simulink model "RadarAltimeter"  (R2020b)
settings: Solver=FixedStepAuto  StartTime=0.0  StopTime=0.0001  FixedStep=T_step  RelTol=1e-3
values from neighbouring files (symbols this model uses):
  BPFden = [RH*RL*CH*CL,RH*CH+RL*CL,1]    [RadarAltEval2.m]
  BPFnum = [RH*CH,0]    [RadarAltEval2.m]
  f_carrier = 1e9    (= 1000000000)    [RadarAltEval.m]    (also in RadarAltEval2.m = 450000000)
  f_square = 500000    [RadarAltEval.m]    (also in RadarAltEval2.m = 250000)
  FMgain = 5    [RadarAltEval.m]    (also in RadarAltEval2.m)
  h = 20    [RadarAltEval.m]    (also in RadarAltEval2.m = 80)
  k_VCO = 2*BW/V_square    (= 200)    [RadarAltEval.m]    (also in RadarAltEval2.m = 400)
  LPFden = conv(LPFden,LPFden)    [RadarAltEval2.m]
  LPFnum = 1    [RadarAltEval2.m]
  noiseVar = 0    [RadarAltEval.m]    (also in RadarAltEval2.m)
  RXdir = 1.76    [RadarAltEval.m]    (also in RadarAltEval2.m)
  RXnoiseVar = 0    [RadarAltEval.m]    (also in RadarAltEval2.m)
  speed = 0    [RadarAltEval.m]    (also in RadarAltEval2.m)
  TXdir = 1.76    [RadarAltEval.m]    (also in RadarAltEval2.m)
  V_square = 10    [RadarAltEval.m]    (also in RadarAltEval2.m)
undefined symbols (not defined in the file or in its folder): magnitude
settings Model: Creator=Joseph  LastModifiedBy=Joseph

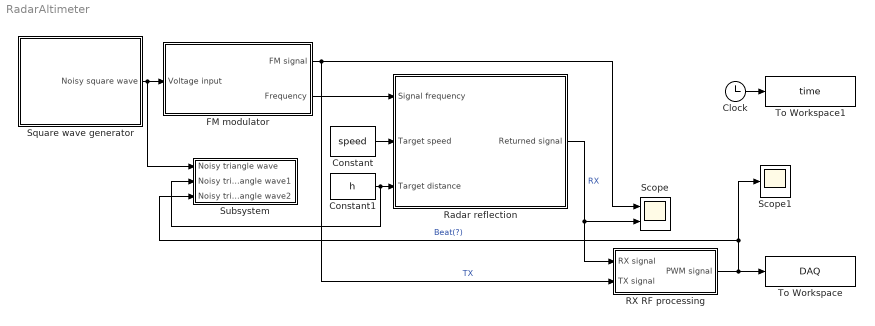
== system RadarAltimeter ==
  Clock : Clock
  Constant : Constant  Value=speed
  Constant1 : Constant  Value=h
  FM modulator : Subsystem
  RX RF processing : Subsystem
  Radar reflection : Subsystem
  Scope : Scope  NumInputPorts=2
  Scope1 : Scope
  Square wave generator : Subsystem
  Subsystem : Subsystem
  To Workspace : ToWorkspace  VariableName=DAQ  SampleTime=-1
  To Workspace1 : ToWorkspace  VariableName=time  SampleTime=-1
  wires:
  Square wave generator/1(Noisy square wave) -> Subsystem/1(Noisy triangle wave), FM modulator/1(Voltage input)
  FM modulator/1(FM signal) -> RX RF processing/2(TX signal), Scope/1  "TX"
  Radar reflection/1(Returned signal) -> RX RF processing/1(RX signal), Scope/2  "RX"
  FM modulator/2(Frequency) -> Radar reflection/1(Signal frequency)
  Constant/1 -> Radar reflection/2(Target speed)
  Constant1/1 -> Subsystem/2(Noisy triangle wave1), Radar reflection/3(Target distance)
  RX RF processing/1(PWM signal) -> Subsystem/3(Noisy triangle wave2), Scope1/1, To Workspace/1  "Beat(?)"
  Clock/1 -> To Workspace1/1

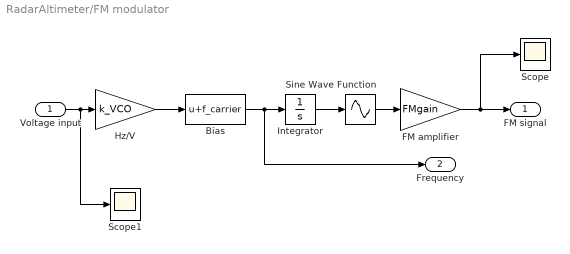
== system RadarAltimeter/FM modulator ==
  Voltage input : Inport
  Bias : Bias  Bias=f_carrier
  FM amplifier : Gain  Gain=FMgain
  Hz/V : Gain  Gain=k_VCO
  Integrator : Integrator
  Scope : Scope
  Scope1 : Scope
  Sine Wave Function : Sin  TimeSource=Use external signal  Frequency=2*pi  SampleTime=0
  FM signal : Outport
  Frequency : Outport  Port=2
  wires:
  Voltage input/1 -> Scope1/1, Hz/V/1
  Sine Wave Function/1 -> FM amplifier/1
  Bias/1 -> Frequency/1, Integrator/1
  Hz/V/1 -> Bias/1
  Integrator/1 -> Sine Wave Function/1
  FM amplifier/1 -> Scope/1, FM signal/1

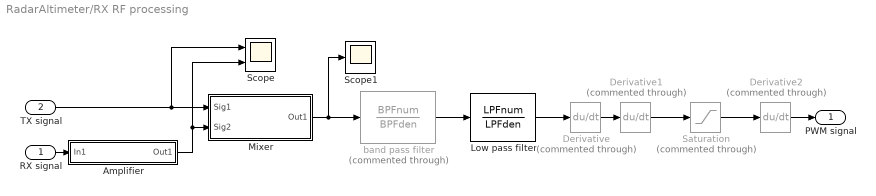
== system RadarAltimeter/RX RF processing ==
  RX signal : Inport
  TX signal : Inport  Port=2
  Amplifier : Subsystem
  Derivative : Derivative  Commented=through
  Derivative1 : Derivative  Commented=through
  Derivative2 : Derivative  Commented=through
  Low pass filter : TransferFcn  Numerator=LPFnum  Denominator=LPFden
  Mixer : Subsystem
  Saturation : Saturate  Commented=through  UpperLimit=3  LowerLimit=0
  Scope : Scope  NumInputPorts=2
  Scope1 : Scope
  band pass filter : TransferFcn  Commented=through  Numerator=BPFnum  Denominator=BPFden
  PWM signal : Outport
  wires:
  TX signal/1 -> Mixer/1(Sig1), Scope/1
  Mixer/1(Out1) -> band pass filter/1, Scope1/1
  Amplifier/1(Out1) -> Scope/2, Mixer/2(Sig2)
  RX signal/1 -> Amplifier/1(In1)
  Derivative/1 -> Derivative1/1
  band pass filter/1 -> Low pass filter/1
  Low pass filter/1 -> Derivative/1
  Saturation/1 -> Derivative2/1
  Derivative1/1 -> Saturation/1
  Derivative2/1 -> PWM signal/1

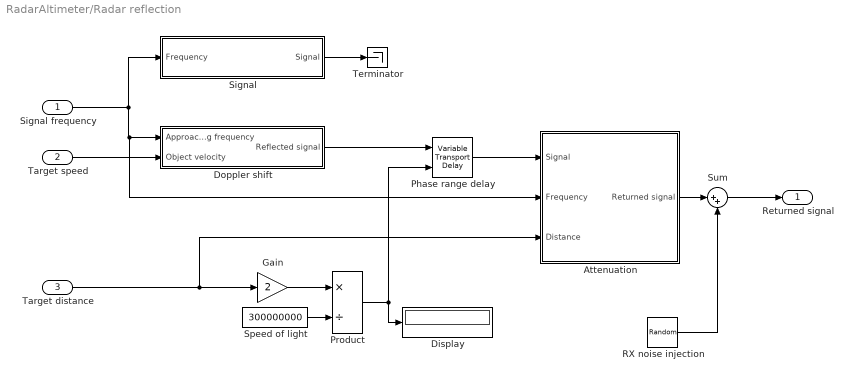
== system RadarAltimeter/Radar reflection ==
  Signal frequency : Inport
  Target speed : Inport  Port=2
  Target distance : Inport  Port=3
  Attenuation : Subsystem
  Display : Display
  Doppler shift : Subsystem
  Gain : Gain  Gain=2
  Phase range delay : VariableTransportDelay  MaximumDelay=10
  Product : Product  Inputs=*/
  RX noise injection : RandomNumber  Variance=RXnoiseVar  Seed=randi([0,10000])  SampleTime=0.1
  Signal : Subsystem
  Speed of light : Constant  Value=300000000
  Sum : Sum  Inputs=|++
  Terminator : Terminator
  Returned signal : Outport
  wires:
  Sum/1 -> Returned signal/1
  Doppler shift/1(Reflected signal) -> Phase range delay/1
  Phase range delay/1 -> Attenuation/1(Signal)
  Signal frequency/1 -> Attenuation/2(Frequency), Doppler shift/1(Approaching frequency), Signal/1(Frequency)
  Gain/1 -> Product/1
  Speed of light/1 -> Product/2
  Product/1 -> Display/1, Phase range delay/2
  Target distance/1 -> Attenuation/3(Distance), Gain/1
  Target speed/1 -> Doppler shift/2(Object velocity)
  Attenuation/1(Returned signal) -> Sum/1
  RX noise injection/1 -> Sum/2
  Signal/1(Signal) -> Terminator/1

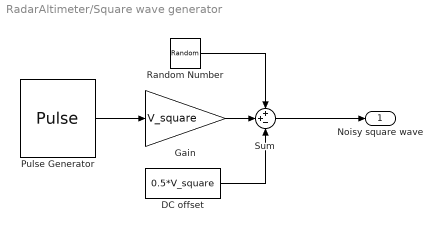
== system RadarAltimeter/Square wave generator ==
  DC offset : Constant  Value=0.5*V_square
  Gain : Gain  Gain=V_square
  Pulse Generator : DiscretePulseGenerator  PulseType=Time based  Period=1/f_square  PulseWidth=50
  Random Number : RandomNumber  Variance=noiseVar  Seed=randi([0,10000])
  Sum : Sum  Inputs=++-
  Noisy square wave : Outport
  wires:
  Pulse Generator/1 -> Gain/1
  Gain/1 -> Sum/2
  DC offset/1 -> Sum/3
  Sum/1 -> Noisy square wave/1
  Random Number/1 -> Sum/1

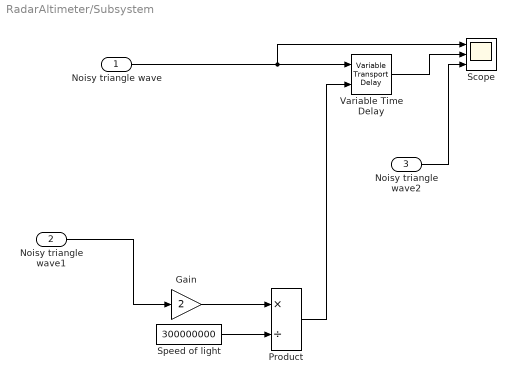
== system RadarAltimeter/Subsystem ==
  Noisy triangle wave : Inport
  Noisy triangle wave1 : Inport  Port=2
  Noisy triangle wave2 : Inport  Port=3
  Gain : Gain  Gain=2
  Product : Product  Inputs=*/
  Scope : Scope  NumInputPorts=3
  Speed of light : Constant  Value=300000000
  Variable Time Delay : VariableTransportDelay  MaximumDelay=10
  wires:
  Noisy triangle wave/1 -> Scope/1, Variable Time Delay/1
  Gain/1 -> Product/1
  Noisy triangle wave1/1 -> Gain/1
  Speed of light/1 -> Product/2
  Product/1 -> Variable Time Delay/2
  Variable Time Delay/1 -> Scope/2
  Noisy triangle wave2/1 -> Scope/3

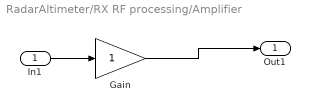
== system RadarAltimeter/RX RF processing/Amplifier ==
  In1 : Inport
  Gain : Gain
  Out1 : Outport
  wires:
  In1/1 -> Gain/1
  Gain/1 -> Out1/1

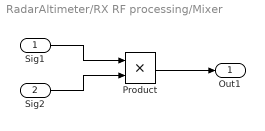
== system RadarAltimeter/RX RF processing/Mixer ==
  Sig1 : Inport
  Sig2 : Inport  Port=2
  Product : Product
  Out1 : Outport
  wires:
  Sig1/1 -> Product/1
  Sig2/1 -> Product/2
  Product/1 -> Out1/1

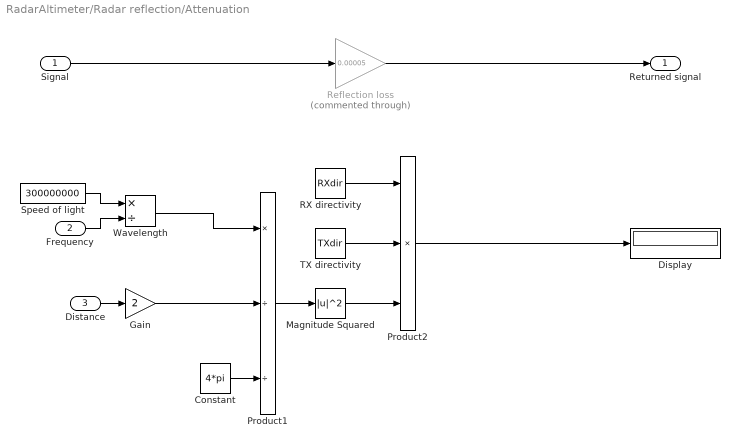
== system RadarAltimeter/Radar reflection/Attenuation ==
  Signal : Inport
  Frequency : Inport  Port=2
  Distance : Inport  Port=3
  Constant : Constant  Value=4*pi
  Display : Display
  Gain : Gain  Gain=2
  Magnitude Squared : Math  Operator=magnitude^2  SaturateOnIntegerOverflow=on
  Product1 : Product  Inputs=*//
  Product2 : Product  Inputs=3
  RX directivity : Constant  Value=RXdir
  Reflection loss : Gain  Commented=through  Gain=0.00005
  Speed of light : Constant  Value=300000000
  TX directivity : Constant  Value=TXdir
  Wavelength : Product  Inputs=*/
  Returned signal : Outport
  wires:
  Signal/1 -> Reflection loss/1
  Distance/1 -> Gain/1
  Speed of light/1 -> Wavelength/1
  Frequency/1 -> Wavelength/2
  Wavelength/1 -> Product1/1
  Gain/1 -> Product1/2
  Constant/1 -> Product1/3
  Product1/1 -> Magnitude Squared/1
  Magnitude Squared/1 -> Product2/3
  TX directivity/1 -> Product2/2
  RX directivity/1 -> Product2/1
  Product2/1 -> Display/1
  Reflection loss/1 -> Returned signal/1

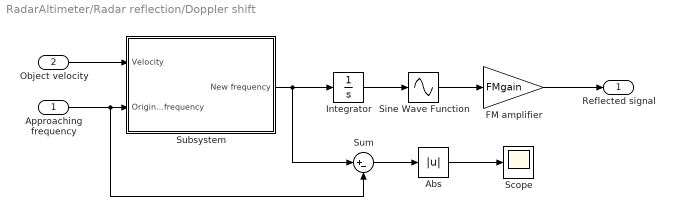
== system RadarAltimeter/Radar reflection/Doppler shift ==
  Approaching frequency : Inport
  Object velocity : Inport  Port=2
  Abs : Abs
  FM amplifier : Gain  Gain=FMgain
  Integrator : Integrator
  Scope : Scope
  Sine Wave Function : Sin  TimeSource=Use external signal  Frequency=2*pi  SampleTime=0
  Subsystem : Subsystem
  Sum : Sum  Inputs=|+-
  Reflected signal : Outport
  wires:
  Approaching frequency/1 -> Sum/2, Subsystem/2(Original frequency)
  Subsystem/1(New frequency) -> Sum/1, Integrator/1
  Integrator/1 -> Sine Wave Function/1
  Sine Wave Function/1 -> FM amplifier/1
  Object velocity/1 -> Subsystem/1(Velocity)
  Sum/1 -> Abs/1
  Abs/1 -> Scope/1
  FM amplifier/1 -> Reflected signal/1

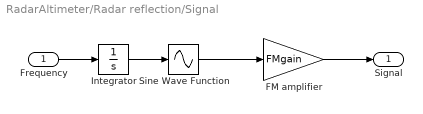
== system RadarAltimeter/Radar reflection/Signal ==
  Frequency : Inport
  FM amplifier : Gain  Gain=FMgain
  Integrator : Integrator
  Sine Wave Function : Sin  TimeSource=Use external signal  Frequency=2*pi  SampleTime=0
  Signal : Outport
  wires:
  Frequency/1 -> Integrator/1
  Integrator/1 -> Sine Wave Function/1
  Sine Wave Function/1 -> FM amplifier/1
  FM amplifier/1 -> Signal/1

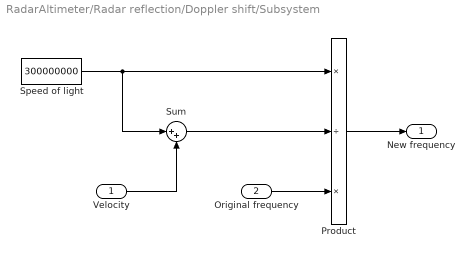
== system RadarAltimeter/Radar reflection/Doppler shift/Subsystem ==
  Velocity : Inport
  Original frequency : Inport  Port=2
  Product : Product  Inputs=*/*
  Speed of light : Constant  Value=300000000
  Sum : Sum  Inputs=|++
  New frequency : Outport
  wires:
  Speed of light/1 -> Sum/1, Product/1
  Product/1 -> New frequency/1
  Original frequency/1 -> Product/3
  Velocity/1 -> Sum/2
  Sum/1 -> Product/2
